simulink model "QUATRE_QUADRANTS"  (R2018a)
settings: Solver=ode45  StartTime=0.0  StopTime=3  RelTol=1e-3  EnableMultiTasking=on
libraries: powerlib x13, powerlib_meascontrol x1
settings Model: Creator=Amal  LastModifiedBy=Utilisateur
settings DataIOCC: LimitDataPoints=on  SaveFormat=Array
settings OptimizationCC: LifeSpan=inf
settings DebuggingCC: UnderspecifiedInitializationDetection=Classic  MergeDetectMultiDrivingBlocksExec=none  SolverPrmCheckMsg=warning  SFUnexpectedBacktrackingDiag=warning  SFNoUnconditionalDefaultTransitionDiag=warning  SFExecutionAtInitializationDiag=none
settings HardwareCC: ProdBitPerPointer=32  ProdBitPerSizeT=32  ProdBitPerPtrDiffT=32  ProdLargestAtomicFloat=None  ProdIntDivRoundTo=Undefined  ProdEndianess=Unspecified  ProdWordSize=32  ProdHWDeviceType=32-bit Generic
settings ModelReferenceCC: PropagateSignalLabelsOutOfModel=off
settings CodeAppCC: StateflowObjectComments=on
settings GRTTargetCC: TargetLangStandard=C89/C90 (ANSI)  GeneratePreprocessorConditionals=Disable all
settings ConfigComp: CovMetricSettings=dw  CovHtmlReporting=on  CovSaveCumulativeToWorkspaceVar=on  CovSaveSingleToWorkspaceVar=on  CovExternalEMLEnable=off
settings SimscapeCC: SimscapeNormalizeSystem=off

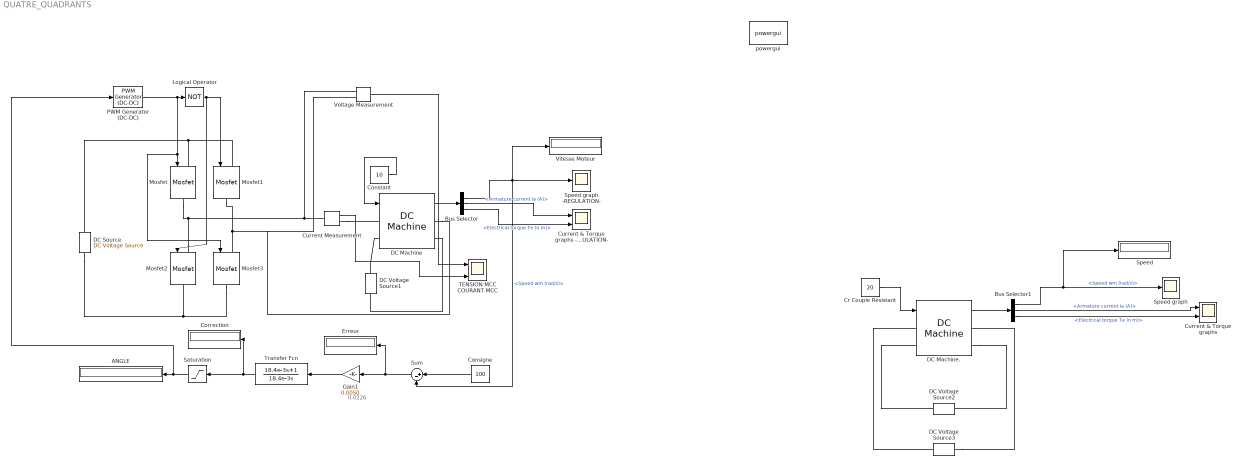
== system QUATRE_QUADRANTS ==
  note: 0.0226
  ANGLE : Display
  Bus Selector : BusSelector  OutputSignals=Speed wm (rad/s),Armature current ia (A),Electrical torque Te (n m)
  Bus Selector1 : BusSelector  OutputSignals=Speed wm (rad/s),Armature current ia (A),Electrical torque Te (n m)
  Consigne : Constant  Value=100
  Constant : Constant  Value=10
  Correction : Display
  Cr Couple Résistant : Constant  Value=20
  "Current & Torque graphs " : Scope  NumInputPorts=2
  Current & Torque graphs -REGULATION- : Scope  NumInputPorts=2
  Current Measurement : powerlib/Measurements/Current Measurement  PhasorSimulation=off  OutputType=Complex  PSBequivalent=0
  DC Machine : powerlib/Machines/DC Machine  PresetModel=02: 5HP 240V 1750RPM Field:150V  MechanicalLoad=Torque TL  FieldType=Wound  ShowDetailedParameters=on  MeasurementBus=off  RLa=[0.78 0.016]  RLf=[150 112.5]  Laf=1.234  MachineConstant=Torque constant (N.m/A)  Ke=1.8  Kt=1.8  J=0.05  Bm=0.01  Tf=0  w0=1  Ifinit=1  TsPowergui=0  TsBlock=-1
  DC Machine. : powerlib/Machines/DC Machine  PresetModel=02: 5HP 240V 1750RPM Field:150V  MechanicalLoad=Torque TL  FieldType=Wound  ShowDetailedParameters=on  MeasurementBus=off  RLa=[0.78 0.016]  RLf=[150 112.5]  Laf=1.234  MachineConstant=Torque constant (N.m/A)  Ke=1.8  Kt=1.8  J=0.05  Bm=0.01  Tf=0  w0=1  Ifinit=1  TsPowergui=0  TsBlock=-1
  DC Source : powerlib/Electrical Sources/DC Voltage Source  Amplitude=240  Measurements=None
  DC Voltage Source1 : powerlib/Electrical Sources/DC Voltage Source  Amplitude=150  Measurements=None
  DC Voltage Source2 : powerlib/Electrical Sources/DC Voltage Source  Amplitude=150  Measurements=None
  DC Voltage Source3 : powerlib/Electrical Sources/DC Voltage Source  Amplitude=240  Measurements=None
  Erreur : Display
  Gain1 : Gain  Gain=0.0050
  Logical Operator : Logic  Operator=NOT  AllPortsSameDT=off  OutDataTypeStr=boolean
  Mosfet{,1..3} (4 alike) : powerlib/Power Electronics/Mosfet  Ron=0.1  Lon=0  Rd=0.01  Vfd=0  IC=0  Rs=1e5  Cs=inf  Measurements=off
  PWM Generator (DC-DC) : powerlib_meascontrol/Pulse & Signal Generators/PWM Generator (DC-DC)  Fsw=2000  Ts=0
  Saturation : Saturate  UpperLimit=1  LowerLimit=0
  Speed : Display
  Speed graph : Scope
  Speed graph -REGULATION- : Scope
  Sum : Sum  Inputs=|+-
  TENSION MCC COURANT MCC : Scope  NumInputPorts=2
  Transfer Fcn : TransferFcn  Numerator=[18.4e-3 1]  Denominator=[18.4e-3 0]
  Vitesse Moteur : Display
  Voltage Measurement : powerlib/Measurements/Voltage Measurement  PhasorSimulation=off  OutputType=Complex  PSBequivalent=0
  powergui : powerlib/powergui  Priority=1  SimulationMode=Continuous  SampleTime=50e-6  frequency=60  Iterations=50  frequencyindice=0  Pbase=100e6  ErrMax=1e-4  UnitsV=kV  UnitsW=MW  buscounter=0  FunctionMessages=off  echomessages=off  EnableUseOfTLC=off  CurrentSourceSwitches=off  DisableSnubberDevices=off  DisableRonSwitches=off  DisableVfSwitches=off  DisplayEquations=off  SolverType=Tustin  Interpol=off  ExternalGateDelay=off  methode=off  Ts=0  x0status=blocks  SPID=off  SwTol=0  HookPort=off  RestoreLinks=warning  ResistiveCurrentMeasurement=off  Frange=[0:2:500]  Ylog=off  Xlog=on  ShowGrid=off  save=off  variable=ZData  structure=0  ZoomFFT=off  StartTime=0.0  cycles=1  DisplayStyle=1  fundamental=60  FreqAxis=off  MaxFrequency=1000  frequencyindicesteady=1  RmsSteady=1  display=off
  wires:
  Constant/1 -> DC Machine/1
  DC Machine/1 -> Bus Selector/1
  Logical Operator/1 -> Mosfet1/1, Mosfet2/1
  Voltage Measurement/1 -> TENSION MCC COURANT MCC/1
  Bus Selector/2 -> Current & Torque graphs -REGULATION-/1  "<Armature current ia (A)>"
  Bus Selector/3 -> Current & Torque graphs -REGULATION-/2  "<Electrical torque Te (n m)>"
  Sum/1 -> Gain1/1, Erreur/1
  PWM Generator (DC-DC)/1 -> Mosfet3/1, Mosfet/1, Logical Operator/1
  Consigne/1 -> Sum/1
  Bus Selector/1 -> Vitesse Moteur/1, Speed graph -REGULATION-/1, Sum/2  "<Speed wm (rad/s)>"
  Saturation/1 -> PWM Generator (DC-DC)/1, ANGLE/1
  Gain1/1 -> Transfer Fcn/1
  Transfer Fcn/1 -> Correction/1, Saturation/1
  Current Measurement/1 -> TENSION MCC COURANT MCC/2
  Cr Couple Résistant/1 -> DC Machine./1
  Bus Selector1/1 -> Speed/1, Speed graph/1  "<Speed wm (rad/s)>"
  Bus Selector1/3 -> "Current & Torque graphs "/2  "<Electrical torque Te (n m)>"
  Bus Selector1/2 -> "Current & Torque graphs "/1  "<Armature current ia (A)>"
  DC Machine./1 -> Bus Selector1/1
  connections:
  Mosfet1/LConn1 -- DC Source/RConn1 -- Mosfet/LConn1
  Mosfet3/LConn1 -- DC Machine/RConn1 -- Voltage Measurement/LConn2 -- Mosfet1/RConn1
  DC Source/LConn1 -- Mosfet3/RConn1 -- Mosfet2/RConn1
  DC Voltage Source1/RConn1 -- DC Machine/LConn2
  DC Machine/RConn2 -- DC Voltage Source1/LConn1
  Voltage Measurement/LConn1 -- Mosfet2/LConn1 -- Mosfet/RConn1 -- Current Measurement/LConn1
  Current Measurement/RConn1 -- DC Machine/LConn1
  DC Machine./LConn2 -- DC Voltage Source2/RConn1
  DC Machine./RConn2 -- DC Voltage Source2/LConn1
  DC Voltage Source3/LConn1 -- DC Machine./RConn1
  DC Voltage Source3/RConn1 -- DC Machine./LConn1
